simulink model "Jan23Lab2model"  (R2012b)
settings: Solver=ode1  StartTime=0.0  StopTime=inf  FixedStep=0.002  RelTol=1e-3
undefined symbols (not defined in the file or in its folder): HIL
libraries: quarc_library x3
settings Model: SimulationMode=external  ExtModeTrigDuration=5000  Creator=crbonney  LastModifiedBy=crbonney
settings SolverCC: PositivePriorityOrder=on
settings RTWCC: SystemTargetFile=quarc_win64.tlc  TemplateMakefile=quarc_default_tmf  Description=QUARC Win64 Target  ProcessScript=quarc_win64_make_rtw_hook
settings STFCustomTargetCC: TargetPreCompLibLocation=C:\PROGRA~3\QUARC\lib\2012b\win64\release  CodeReplacementLibrary=ANSI_C  GeneratePreprocessorConditionals=Disable all  CombineOutputUpdateFcns=on  GRTInterface=off  SystemTargetFile=quarc_win64.tlc
settings GRTTargetCC: TargetPreCompLibLocation=C:\PROGRA~3\QUARC\lib\2012b\win64\release  ParMdlRefBuildCompliant=off  CompOptLevelCompliant=off  ConcurrentExecutionCompliant=off  MatFileLogging=off  ExtMode=on  ExtModeMexFile=quarc_comm

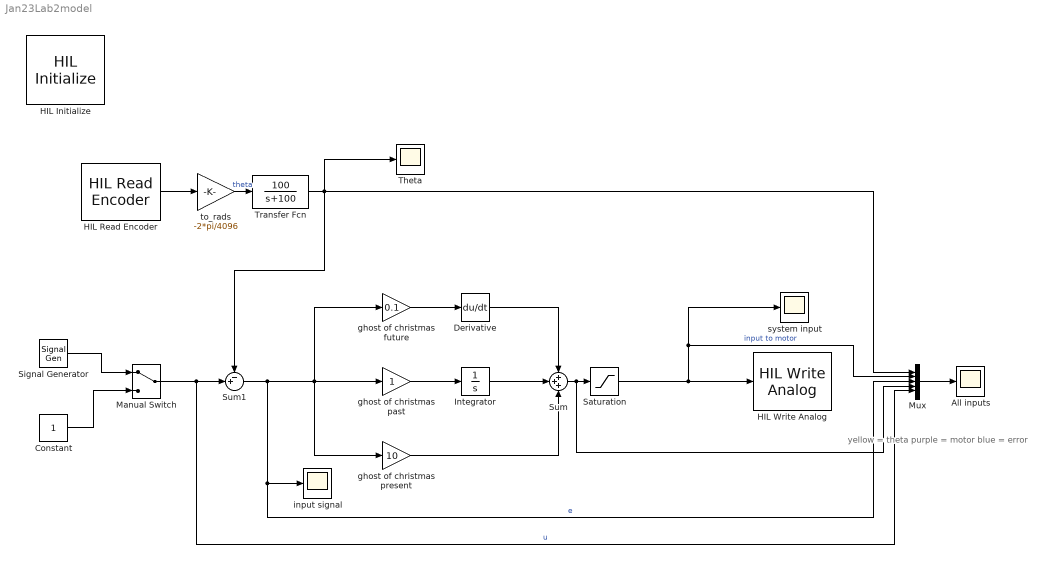
== system Jan23Lab2model ==
  note: yellow = theta
      | purple = motor
      | blue = error
  All inputs : Scope
      settings: YMin=-5.5  YMax=2.5  SaveName=ScopeData4
  Constant : Constant
  Derivative : Derivative
  HIL Initialize : quarc_library/Data Acquisition/Generic/Configuration/HIL Initialize  Priority=-99  object_name=HIL-1  board_type=q2_usb  board_number=0  board_options=d0=digital;d1=digital;led=auto;update_rate=normal;decimation=1  exclusive=off  active=off  hardware_clocks=[0]  clock_modes=[]  initial_clock_frequencies=[]  set_clock_params_at_start=off  set_clock_params_at_switch_in=off  set_clock_frequencies_at_start=off  set_clock_frequencies_at_switch_in=off  analog_input_channels=[0:1]  analog_input_maximums=10  analog_input_minimums=-10  set_analog_input_params_at_start=on  set_analog_input_params_at_switch_in=off  analog_output_channels=[0:1]  analog_output_maximums=10  analog_output_minimums=-10  initial_analog_outputs=[0]  final_analog_outputs=[0]  watchdog_analog_outputs=0  set_analog_output_params_at_start=on  set_analog_output_params_at_switch_in=off  set_analog_outputs_at_start=on  set_analog_outputs_at_switch_in=off  set_analog_outputs_at_terminate=on  set_analog_outputs_at_switch_out=off  set_analog_outputs_on_watchdog=off  digital_input_channels=[]  digital_output_channels=[]  digital_output_configuration=[]  initial_digital_outputs=[1]  final_digital_outputs=[1]  watchdog_digital_outputs=[1]  set_digital_output_params_at_start=off  set_digital_output_params_at_switch_in=off  set_digital_outputs_at_start=on  set_digital_outputs_at_switch_in=off  set_digital_outputs_at_terminate=on  set_digital_outputs_at_switch_out=off  set_digital_outputs_on_watchdog=off  encoder_channels=[0:1]  quadrature=[4]  encoder_filter_frequency=[]  initial_encoder_counts=[0]  set_encoder_params_at_start=on  set_encoder_params_at_switch_in=off  set_encoder_counts_at_start=on  set_encoder_counts_at_switch_in=off  pwm_channels=[]  pwm_modes=[0]  pwm_frequency=1/0.020  pwm_configuration=[]  pwm_alignment=[]  pwm_polarity=[]  pwm_leading_deadband=[]  pwm_trailing_deadband=[]  initial_pwm_outputs=[0]  final_pwm_outputs=[0]  watchdog_pwm_outputs=[0]  set_pwm_params_at_start=on  set_pwm_params_at_switch_in=off  set_pwm_outputs_at_start=on  set_pwm_outputs_at_switch_in=off  set_pwm_outputs_at_terminate=on  set_pwm_outputs_at_switch_out=off  set_pwm_outputs_on_watchdog=off  other_output_channels=[]  initial_other_outputs=[]  final_other_outputs=[]  watchdog_other_outputs=[]  set_other_outputs_at_start=off  set_other_outputs_at_switch_in=off  set_other_outputs_at_terminate=off  set_other_outputs_at_switch_out=off  set_other_outputs_on_watchdog=off
  HIL Read Encoder : quarc_library/Data Acquisition/Generic/Immediate I//O/HIL Read Encoder  object_name=HIL-1  channels=0  sample_time=qc_get_step_size  active=on  vector_output=off  data_type_mode=Inherit via back propagation  data_type=double
  HIL Write Analog : quarc_library/Data Acquisition/Generic/Immediate I//O/HIL Write Analog  object_name=HIL-1  channels=0  sample_time=-1  active=off  vector_input=off
  Integrator : Integrator
  Manual Switch : ManualSwitch
  Mux : Mux  Inputs=5
  Saturation : Saturate  UpperLimit=10  LowerLimit=-10
  Signal Generator : SignalGenerator  WaveForm=square  Frequency=.1
  Sum : Sum  Inputs=+++
  Sum1 : Sum  Inputs=-+|
  Theta : Scope
      settings: YMin=-0.45  YMax=0.45
  Transfer Fcn : TransferFcn  Numerator=[100]  Denominator=[1 100]
  ghost of christmas future : Gain  Gain=0.1
      settings: AttributesFormatString=k=%<Gain>
  ghost of christmas past : Gain
      settings: AttributesFormatString=k=%<Gain>
  ghost of christmas present : Gain  Gain=10
      settings: AttributesFormatString=k=%<Gain>
  input signal : Scope
      settings: YMin=-1.75  YMax=1.75  SaveName=ScopeData3
  system input : Scope
      settings: YMin=-1.75  YMax=1.75
  to_rads : Gain  Gain=-2*pi/4096
  wires:
  to_rads/1 -> Transfer Fcn/1  "theta"
  HIL Read Encoder/1 -> to_rads/1
  ghost of christmas past/1 -> Integrator/1
  Integrator/1 -> Sum/2
  Derivative/1 -> Sum/1
  ghost of christmas present/1 -> Sum/3
  Sum1/1 -> input signal/1, Mux/3, ghost of christmas past/1, ghost of christmas future/1, ghost of christmas present/1  "e"
  Manual Switch/1 -> Mux/5, Sum1/2  "u"
  Saturation/1 -> HIL Write Analog/1, Mux/2, system input/1  "input to motor"
  ghost of christmas future/1 -> Derivative/1
  Mux/1 -> All inputs/1
  Transfer Fcn/1 -> Mux/1, Theta/1, Sum1/1
  Sum/1 -> Mux/4, Saturation/1
  Constant/1 -> Manual Switch/2
  Signal Generator/1 -> Manual Switch/1
